simulink model "testEnabledSubsystem"  (R2014a)
settings: Solver=FixedStepDiscrete  StartTime=0.0  StopTime=Inf  FixedStep=0.001  RelTol=1e-3
libraries: libButtons x1
settings Model: Creator=shenoylab  LastModifiedBy=shenoylab

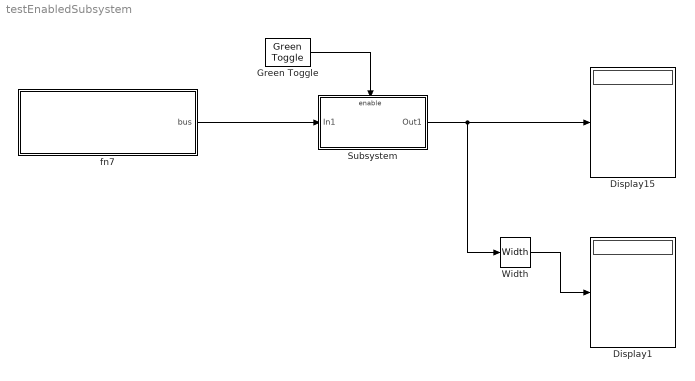
== system testEnabledSubsystem ==
  Display1 : Display
  Display15 : Display
  Green Toggle : libButtons/Green Toggle  SystemSampleTime=-1
  Subsystem : Subsystem
  Width : Width
  fn7 : MATLAB Function  TreatAsAtomicUnit=on
  wires:
  fn7/1(bus) -> Subsystem/1(In1)
  Subsystem/1(Out1) -> Width/1, Display15/1
  Width/1 -> Display1/1
  Green Toggle/1 -> Subsystem/Enable

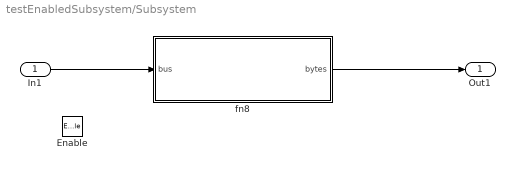
== system testEnabledSubsystem/Subsystem ==
  In1 : Inport
  Enable : EnablePort  StatesWhenEnabling=reset  PropagateVarSize=During execution
  fn8 : MATLAB Function  TreatAsAtomicUnit=on
  Out1 : Outport  OutputWhenDisabled=reset
  wires:
  In1/1 -> fn8/1(bus)
  fn8/1(bytes) -> Out1/1

== matlab function testEnabledSubsystem/fn7 ==
  data: bus output Bus: TestBusOuter size=1
function bus = createBus()

bus = testSerializedParamsLib.initializeBus_TestBusOuter();
P1 = testSerializedParamsLib.initializeBus_TestBusInner();

P1.centerSize = uint8([1 2])';
P1.holdWindowCenter = uint8(2);
P1.holdWindowTarget = uint16(30);

bus.val1 = uint8(3);
bus.val2 = uint8('hello')';
bus.valEnum = TestEnum.eval3_longer;
bus.nested = P1;

== matlab function testEnabledSubsystem/Subsystem/fn8 ==
  data: bus input Bus: TestBusOuter size=1; bytes output uint8 size=300
function bytes = serialize(bus)
%#codegen

bytes = testSerializedParamsLib.serializeBus_TestBusOuter(bus);
